simulink model "mission_server_waypoint_qball2"  (Simulink 8.3)
settings: Solver=FixedStepDiscrete  StartTime=0.0  StopTime=inf  FixedStep=0.002  RelTol=1e-3
libraries: quarc_library x6, Orientation_Library x2, simulink x1
settings Model: Creator=CFulford  LastModifiedBy=user  SimulationMode=external  ExtModeTrigDuration=5000
settings SolverCC: PositivePriorityOrder=on
settings OptimizationCC: ExpressionDepthLimit=2147483647  InitFltsAndDblsToZero=on
settings DebuggingCC: FcnCallInpInsideContextMsg=UseLocalSettings
settings SFSimCC: SimParseCustomCode=off
settings RTWCC: SystemTargetFile=quarc_win64.tlc  TemplateMakefile=quarc_default_tmf  Description=QUARC Win64 Target  ProcessScript=quarc_win64_make_rtw_hook
settings STFCustomTargetCC: TargetPreCompLibLocation=C:\PROGRA~3\QUARC\lib\2014a\win64\release  CodeReplacementLibrary=C89/C90 (ANSI)  ConcurrentExecutionCompliant=on  GeneratePreprocessorConditionals=Disable all  CombineOutputUpdateFcns=on  CPPClassGenCompliant=on  GRTInterface=off  SystemTargetFile=quarc_win64.tlc
settings GRTTargetCC: TargetPreCompLibLocation=C:\PROGRA~3\QUARC\lib\2014a\win64\release  CodeReplacementLibrary=C89/C90 (ANSI)  ParMdlRefBuildCompliant=off  CompOptLevelCompliant=off  CombineOutputUpdateFcns=on  MatFileLogging=off  GRTInterface=off  ExtMode=on  ExtModeMexFile=quarc_comm  ExtModeMexArgs='-w -d %d -uri %u','shmem://%m:1?timeout=10'

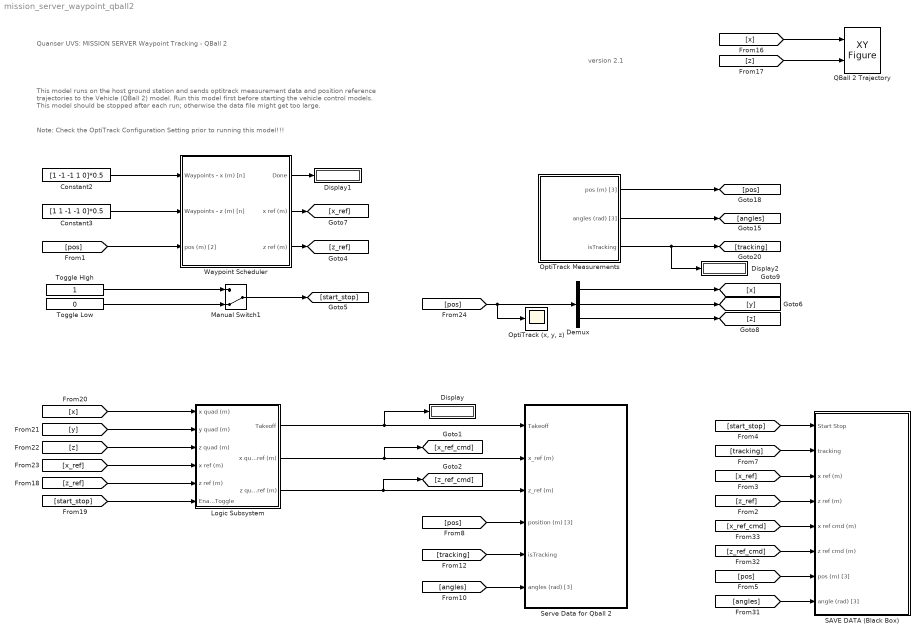
== system mission_server_waypoint_qball2 ==
  note: version 2.1
  note: This model runs on the host ground station and sends
      | optitrack measurement data and position reference trajectories to the Vehicle (QBall 2) model.
      | Run this model first before starting the vehicle control models.
      | This model should be stopped after each run; otherwise the data file might get too large.
  note: Quanser UVS: MISSION SERVER Waypoint Tracking - QBall 2
  note: Note: Check the OptiTrack Configuration Setting prior to running this model!!!
  Constant2 : Constant  Value=[1 -1 -1 1 0]*0.5
  Constant3 : Constant  Value=[1 1 -1 -1 0]*0.5
  Demux : Demux  Outputs=3
  Display : Display
  Display1 : Display
  Display2 : Display
  Logic Subsystem : Subsystem
  Manual Switch1 : ManualSwitch  CurrentSetting=0
  "OptiTrack (x, y, z)" : Scope
      settings: YMin=-0.1  YMax=1.05
  OptiTrack Measurements : Subsystem
  QBall 2 Trajectory : quarc_library/Sinks/Figures/XY Figure  figure_mode=Use figure window  figure_tag=figure1  axes_tag=axes1  minimum_x=-1  maximum_x=1  minimum_y=-1  maximum_y=1  trace_mode=Do not erase old trace  buffer_size=1000  update_rate=100  initial_position="601   63  713  540"  initial_visibility=off  sample_time=-1
  SAVE DATA (Black Box) : Subsystem
  Serve Data for Qball 2 : Subsystem
  Toggle High : Constant
  Toggle Low : Constant  Value=0
  Waypoint Scheduler : Subsystem
  wires:
  [x] -> QBall 2 Trajectory/1
  [z] -> QBall 2 Trajectory/2
  Toggle High/1 -> Manual Switch1/1
  Toggle Low/1 -> Manual Switch1/2
  Manual Switch1/1 -> [start_stop]
  [start_stop] -> Logic Subsystem/6(Enable Toggle)
  [x] -> Logic Subsystem/1(x quad (m))
  [z_ref] -> Logic Subsystem/5(z ref (m))
  [y] -> Logic Subsystem/2(y quad (m))
  [z] -> Logic Subsystem/3(z quad (m))
  [x_ref] -> Logic Subsystem/4(x ref (m))
  Demux/1 -> [x]
  Demux/2 -> [y]
  Demux/3 -> [z]
  OptiTrack Measurements/1(pos (m) [3]) -> [pos]
  OptiTrack Measurements/2(angles (rad) [3]) -> [angles]
  [pos] -> "OptiTrack (x, y, z)"/1, Demux/1
  Logic Subsystem/3(z quad ref (m)) -> [z_ref_cmd], Serve Data for Qball 2/3(z_ref (m))
  Logic Subsystem/1(Takeoff) -> Display/1, Serve Data for Qball 2/1(Takeoff)
  Logic Subsystem/2(x quad ref (m)) -> [x_ref_cmd], Serve Data for Qball 2/2(x_ref (m))
  [tracking] -> Serve Data for Qball 2/5(isTracking)
  [angles] -> Serve Data for Qball 2/6(angles (rad) [3])
  [pos] -> Serve Data for Qball 2/4(position (m) [3])
  OptiTrack Measurements/3(isTracking) -> Display2/1, [tracking]
  Constant3/1 -> Waypoint Scheduler/2(Waypoints - z (m) [n])
  Constant2/1 -> Waypoint Scheduler/1(Waypoints - x (m) [n])
  Waypoint Scheduler/1(Done) -> Display1/1
  Waypoint Scheduler/3(z ref (m)) -> [z_ref]
  Waypoint Scheduler/2(x ref (m)) -> [x_ref]
  [pos] -> Waypoint Scheduler/3(pos (m) [2])
  [z_ref] -> SAVE DATA (Black Box)/4(z ref (m))
  [start_stop] -> SAVE DATA (Black Box)/1(Start Stop)
  [x_ref] -> SAVE DATA (Black Box)/3(x ref (m))
  [pos] -> SAVE DATA (Black Box)/7(pos (m) [3])
  [angles] -> SAVE DATA (Black Box)/8(angle (rad) [3])
  [tracking] -> SAVE DATA (Black Box)/2(tracking)
  [z_ref_cmd] -> SAVE DATA (Black Box)/6(z ref cmd (m))
  [x_ref_cmd] -> SAVE DATA (Black Box)/5(x ref cmd (m))

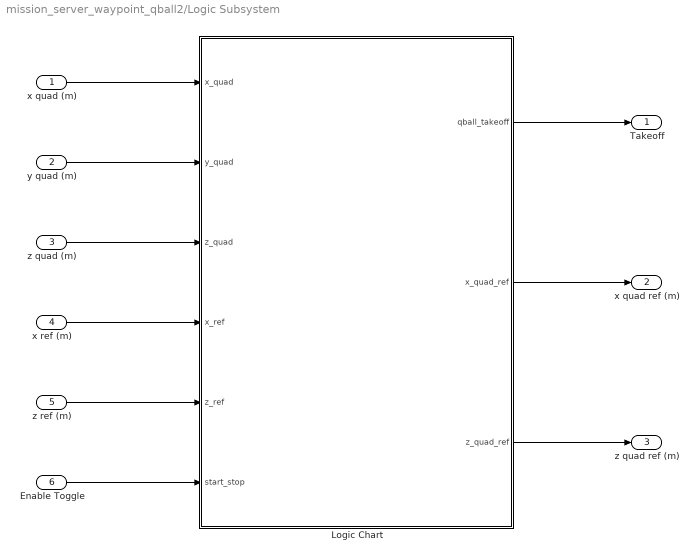
== system mission_server_waypoint_qball2/Logic Subsystem ==
  x quad (m) : Inport
  y quad (m) : Inport  Port=2
  z quad (m) : Inport  Port=3
  x ref (m) : Inport  Port=4
  z ref (m) : Inport  Port=5
  Enable Toggle : Inport  Port=6
  Logic Chart : Stateflow chart  TreatAsAtomicUnit=on
  Takeoff : Outport
  x quad ref (m) : Outport  Port=2
  z quad ref (m) : Outport  Port=3
  wires:
  Logic Chart/2(x_quad_ref) -> x quad ref (m)/1
  Logic Chart/1(qball_takeoff) -> Takeoff/1
  Logic Chart/3(z_quad_ref) -> z quad ref (m)/1
  x quad (m)/1 -> Logic Chart/1(x_quad)
  y quad (m)/1 -> Logic Chart/2(y_quad)
  z quad (m)/1 -> Logic Chart/3(z_quad)
  Enable Toggle/1 -> Logic Chart/6(start_stop)
  x ref (m)/1 -> Logic Chart/4(x_ref)
  z ref (m)/1 -> Logic Chart/5(z_ref)

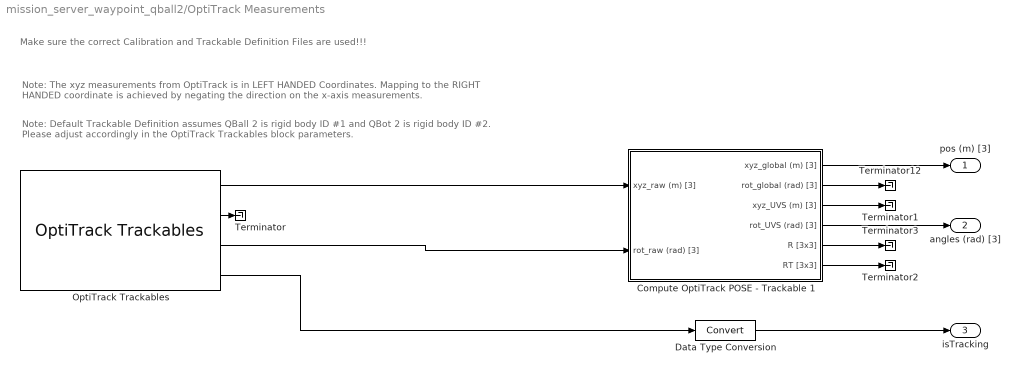
== system mission_server_waypoint_qball2/OptiTrack Measurements ==
  note: Note: The xyz measurements from OptiTrack is in LEFT HANDED Coordinates.
      |
      | Mapping to the RIGHT HANDED coordinate is achieved by negating the direction on the x-axis measurements.
  note: Make sure the correct Calibration and Trackable Definition Files are used!!!
  note: Note: Default Trackable Definition assumes QBall 2 is rigid body ID #1 and QBot 2 is rigid body ID #2.
      | Please adjust accordingly in the OptiTrack Trackables block parameters.
  "Compute OptiTrack POSE - Trackable 1 " : Subsystem
  Data Type Conversion : DataTypeConversion
  OptiTrack Trackables : quarc_library/Devices/Third-Party/NaturalPoint/OptiTrack/OptiTrack Trackables  calibration_file=C:\Users\user\Desktop\final\Calibration Very High Quality Exceptional (MeanErr 0.001 mm) 2017-05-16 6.48pm.cal  rigid_body_file=C:\Users\user\Desktop\final\RigidBodies 2017-05-26 7.29pm.tra  rigid_body_ids=[1]  sample_time=qc_get_step_size
  Terminator{,1..3,12} (5 alike) : Terminator
  pos (m) [3] : Outport
  angles (rad) [3] : Outport  Port=2
  isTracking : Outport  Port=3
  wires:
  OptiTrack Trackables/4 -> Data Type Conversion/1
  OptiTrack Trackables/2 -> Terminator/1
  "Compute OptiTrack POSE - Trackable 1 "/1(xyz_global (m) [3]) -> pos (m) [3]/1
  "Compute OptiTrack POSE - Trackable 1 "/4(rot_UVS (rad) [3]) -> angles (rad) [3]/1
  "Compute OptiTrack POSE - Trackable 1 "/3(xyz_UVS (m) [3]) -> Terminator1/1
  "Compute OptiTrack POSE - Trackable 1 "/2(rot_global (rad) [3]) -> Terminator12/1
  "Compute OptiTrack POSE - Trackable 1 "/5(R [3x3]) -> Terminator3/1
  "Compute OptiTrack POSE - Trackable 1 "/6(RT [3x3]) -> Terminator2/1
  OptiTrack Trackables/1 -> "Compute OptiTrack POSE - Trackable 1 "/1(xyz_raw (m) [3])
  OptiTrack Trackables/3 -> "Compute OptiTrack POSE - Trackable 1 "/2(rot_raw (rad) [3])
  Data Type Conversion/1 -> isTracking/1

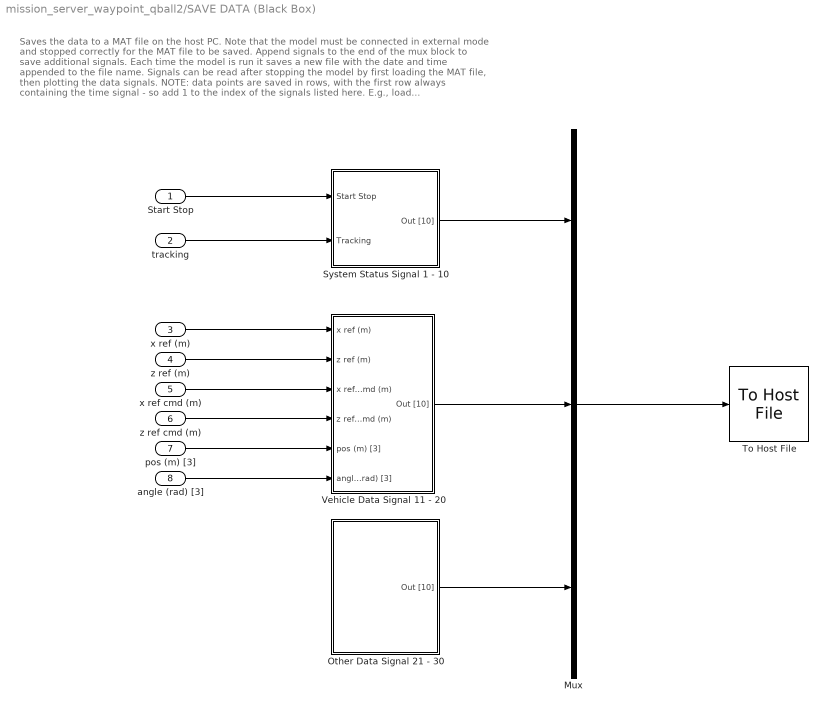
== system mission_server_waypoint_qball2/SAVE DATA (Black Box) ==
  note: Saves the data to a MAT file on the host PC. Note that the model must be connected
      | in external mode and stopped correctly for the MAT file to be saved.
      | Append signals to the end of the mux block to save additional signals.
      | Each time the model is run it saves a new file with the date and time appended
      | to the file name.
      |
      | Signals can be read after stopping the model by first loading the MAT file, then plotting
      | the data signals. NOTE: data points are saved in rows, with the first row always containing
      | the time signal - so add 1 to the index of the signals listed here. E.g.,
      |
      | load mission_data.mat
      | t = mission_data(1,:);
      | roll = mission_data(22,:);
      | plot(t, roll);
  Start Stop : Inport
  tracking : Inport  Port=2
  x ref (m) : Inport  Port=3
  z ref (m) : Inport  Port=4
  x ref cmd (m) : Inport  Port=5
  z ref cmd (m) : Inport  Port=6
  pos (m) [3] : Inport  Port=7
  angle (rad) [3] : Inport  Port=8
  Mux : Mux  Inputs=3
  Other Data Signal 21 - 30 : Subsystem
  System Status Signal 1 - 10 : Subsystem
  To Host File : quarc_library/Sinks/To Host/To Host File  file_name=mission_data_%{date}_%{time}.mat  variable_name=mission_data  decimation=1  sample_time=-1  file_format=MAT-file v.4  options=No header or footer  append=off  final_file_name=mission_data_26-May-2017_19-37-20.mat
  Vehicle Data Signal 11 - 20 : Subsystem
  wires:
  Start Stop/1 -> System Status Signal 1 - 10/1(Start Stop)
  tracking/1 -> System Status Signal 1 - 10/2(Tracking)
  z ref (m)/1 -> Vehicle Data Signal 11 - 20/2(z ref (m))
  x ref (m)/1 -> Vehicle Data Signal 11 - 20/1(x ref (m))
  pos (m) [3]/1 -> Vehicle Data Signal 11 - 20/5(pos (m) [3])
  angle (rad) [3]/1 -> Vehicle Data Signal 11 - 20/6(angle (rad) [3])
  System Status Signal 1 - 10/1(Out [10]) -> Mux/1
  Vehicle Data Signal 11 - 20/1(Out [10]) -> Mux/2
  Other Data Signal 21 - 30/1(Out [10]) -> Mux/3
  Mux/1 -> To Host File/1
  z ref cmd (m)/1 -> Vehicle Data Signal 11 - 20/4(z ref cmd (m))
  x ref cmd (m)/1 -> Vehicle Data Signal 11 - 20/3(x ref cmd (m))

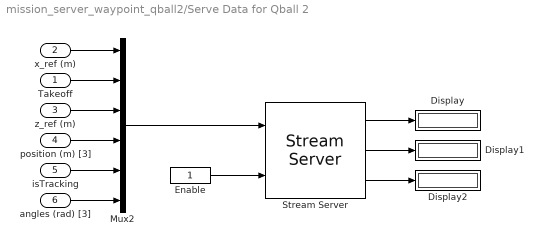
== system mission_server_waypoint_qball2/Serve Data for Qball 2 ==
  Takeoff : Inport
  x_ref (m) : Inport  Port=2
  z_ref (m) : Inport  Port=3
  position (m) [3] : Inport  Port=4
  isTracking : Inport  Port=5
  angles (rad) [3] : Inport  Port=6
  Display : Display
      settings: Decimation=100
  Display1 : Display
      settings: Decimation=100
  Display2 : Display
      settings: Decimation=100
  Enable : Constant
  Mux2 : Mux  Inputs=[1 1 1 3 1 3]
  Stream Server : quarc_library/Communications/Basic/Stream Server  uri_source=Specify via dialog (do not evaluate)  uri=tcpip://localhost:18006  apply_uri_to_all_configs=on  send_buffer_size=1460  receive_buffer_size=1460  byte_order=little endian (Intel - LSB first)  optimization=Minimum latency  implementation=Use non-blocking I/O  send_options=Send most recent data  receive_options=Do not receive data  send_fifo_size=1000  receive_fifo_size=1000  send_priority=0  receive_priority=0  default_value=[0]  send_dimensions=off  receive_dimensions=off  max_dimensions=-1  sample_time=qc_get_step_size  active=off  data_type=Inherited via back propagation  type_expr=BusObject
      settings: AttributesFormatString="\"tcpip://localhost:18006\""
  wires:
  Enable/1 -> Stream Server/2
  Stream Server/1 -> Display/1
  Stream Server/2 -> Display1/1
  Stream Server/3 -> Display2/1
  z_ref (m)/1 -> Mux2/3
  position (m) [3]/1 -> Mux2/4
  Takeoff/1 -> Mux2/2
  isTracking/1 -> Mux2/5
  x_ref (m)/1 -> Mux2/1
  angles (rad) [3]/1 -> Mux2/6
  Mux2/1 -> Stream Server/1

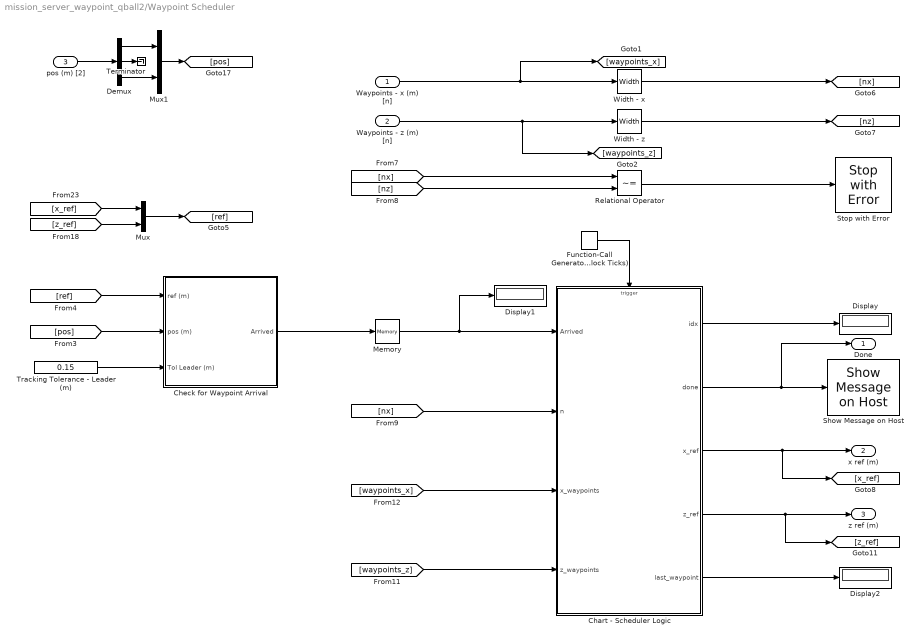
== system mission_server_waypoint_qball2/Waypoint Scheduler ==
  Waypoints - x (m) [n] : Inport
  Waypoints - z (m) [n] : Inport  Port=2
  pos (m) [2] : Inport  Port=3
  Chart - Scheduler Logic : Stateflow chart  TreatAsAtomicUnit=on
  Check for Waypoint Arrival : Subsystem
  Demux : Demux  Outputs=3
  Display : Display
      settings: Decimation=100
  Display1 : Display
      settings: Decimation=100
  Display2 : Display
      settings: Decimation=100
  Function-Call Generator (Clock Ticks) : simulink/Ports & Subsystems/Function-Call Generator  sample_time=qc_get_step_size  numberOfIterations=1
  Memory : Memory
  Mux : Mux  Inputs=2
  Mux1 : Mux  Inputs=2
  Relational Operator : RelationalOperator  Operator=~=  OutDataTypeStr=boolean
  Show Message on Host : quarc_library/Sinks/Error Handling/Show Message on Host  message_type=Fixed error message  message_icon=Information  message=Vehicles at final waypoint. Please land QBall and then stop all models.
      settings: AttributesFormatString="\"%<message>\""
  Stop with Error : quarc_library/Sinks/Error Handling/Stop with Error  message_type=Fixed error message  message=Error: Number of x and z waypoints not equal!
      settings: AttributesFormatString="\"%<message>\""
  Terminator : Terminator
  Tracking Tolerance - Leader (m) : Constant  Value=0.15
  Width - x : Width
  Width - z : Width
  Done : Outport
  x ref (m) : Outport  Port=2
  z ref (m) : Outport  Port=3
  wires:
  Waypoints - x (m) [n]/1 -> Width - x/1, [waypoints_x]
  Waypoints - z (m) [n]/1 -> Width - z/1, [waypoints_z]
  [x_ref] -> Mux/1
  [z_ref] -> Mux/2
  Mux/1 -> [ref]
  Width - x/1 -> [nx]
  Width - z/1 -> [nz]
  [nx] -> Relational Operator/1
  [nz] -> Relational Operator/2
  Relational Operator/1 -> Stop with Error/1
  Chart - Scheduler Logic/3(x_ref) -> [x_ref], x ref (m)/1
  Chart - Scheduler Logic/4(z_ref) -> [z_ref], z ref (m)/1
  Chart - Scheduler Logic/2(done) -> Done/1, Show Message on Host/1
  Chart - Scheduler Logic/1(idx) -> Display/1
  Function-Call Generator (Clock Ticks)/1 -> Chart - Scheduler Logic/Trigger
  [nx] -> Chart - Scheduler Logic/2(n)
  [waypoints_x] -> Chart - Scheduler Logic/3(x_waypoints)
  [waypoints_z] -> Chart - Scheduler Logic/4(z_waypoints)
  [ref] -> Check for Waypoint Arrival/1(ref (m))
  [pos] -> Check for Waypoint Arrival/2(pos (m))
  Check for Waypoint Arrival/1(Arrived) -> Memory/1
  Memory/1 -> Display1/1, Chart - Scheduler Logic/1(Arrived)
  pos (m) [2]/1 -> Demux/1
  Demux/1 -> Mux1/1
  Demux/3 -> Mux1/2
  Mux1/1 -> [pos]
  Demux/2 -> Terminator/1
  Tracking Tolerance - Leader (m)/1 -> Check for Waypoint Arrival/3(Tol Leader (m))
  Chart - Scheduler Logic/5(last_waypoint) -> Display2/1

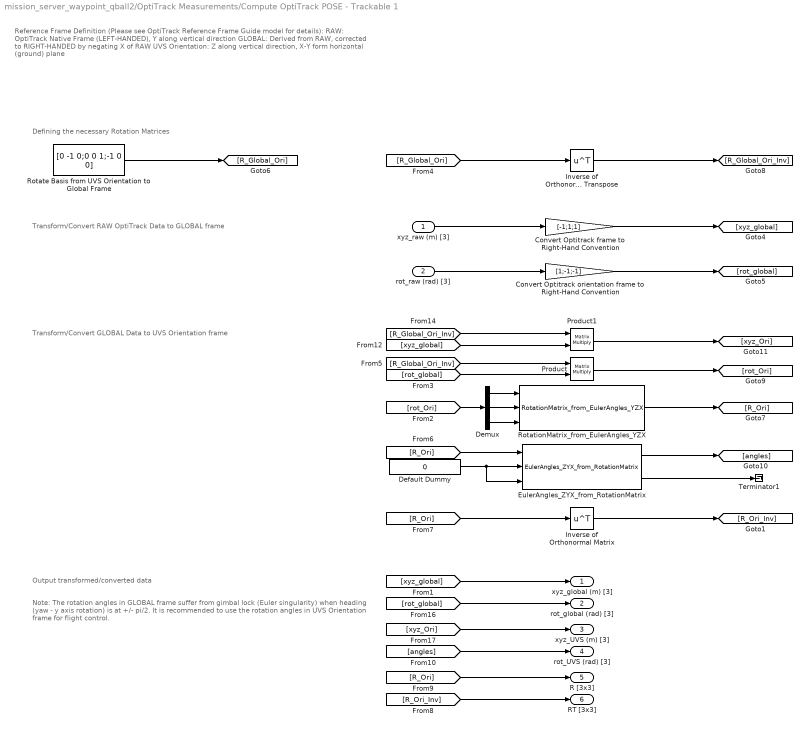
== system mission_server_waypoint_qball2/OptiTrack Measurements/Compute OptiTrack POSE - Trackable 1  ==
  note: Transform/Convert RAW OptiTrack Data to GLOBAL frame
  note: Defining the necessary Rotation Matrices
  note: Reference Frame Definition (Please see OptiTrack Reference Frame Guide model for details):
      |
      | RAW: OptiTrack Native Frame (LEFT-HANDED), Y along vertical direction
      | GLOBAL: Derived from RAW, corrected to RIGHT-HANDED by negating X of RAW
      | UVS Orientation: Z along vertical direction, X-Y form horizontal (ground) plane
  note: Transform/Convert GLOBAL Data to UVS Orientation frame
  note: Output transformed/converted data
  note: Note: The rotation angles in GLOBAL frame suffer from gimbal lock (Euler singularity)
      | when heading (yaw - y axis rotation) is at +/- pi/2.
      | It is recommended to use the rotation angles in UVS Orientation frame for flight control.
  xyz_raw (m) [3] : Inport
  rot_raw (rad) [3] : Inport  Port=2
  Convert Optitrack frame to Right-Hand Convention : Gain  Gain=[-1;1;1]
  Convert Optitrack orientation frame to Right-Hand Convention : Gain  Gain=[1;-1;-1]
  Default Dummy : Constant  Value=0
  Demux : Demux  Outputs=3
  EulerAngles_ZYX_from_RotationMatrix : Orientation_Library/EulerAngles_ZYX_from_RotationMatrix
  Inverse of Orthonormal Matrix : Math  Operator=transpose  SaturateOnIntegerOverflow=on
  Inverse of Orthonormal Matrix is its Transpose : Math  Operator=transpose  SaturateOnIntegerOverflow=on
  Product : Product  Multiplication=Matrix(*)
  Product1 : Product  Multiplication=Matrix(*)
  Rotate Basis from UVS Orientation to Global Frame : Constant  Value=[0 -1 0;0 0 1;-1 0 0]
  RotationMatrix_from_EulerAngles_YZX : Orientation_Library/RotationMatrix_from_EulerAngles_YZX
  Terminator1 : Terminator
  xyz_global (m) [3] : Outport
  rot_global (rad) [3] : Outport  Port=2
  xyz_UVS (m) [3] : Outport  Port=3
  rot_UVS (rad) [3] : Outport  Port=4
  R [3x3] : Outport  Port=5
  RT [3x3] : Outport  Port=6
  wires:
  Rotate Basis from UVS Orientation to Global Frame/1 -> [R_Global_Ori]
  [R_Global_Ori] -> Inverse of Orthonormal Matrix is its Transpose/1
  Inverse of Orthonormal Matrix is its Transpose/1 -> [R_Global_Ori_Inv]
  Convert Optitrack orientation frame to Right-Hand Convention/1 -> [rot_global]
  xyz_raw (m) [3]/1 -> Convert Optitrack frame to Right-Hand Convention/1
  Convert Optitrack frame to Right-Hand Convention/1 -> [xyz_global]
  rot_raw (rad) [3]/1 -> Convert Optitrack orientation frame to Right-Hand Convention/1
  [R_Global_Ori_Inv] -> Product1/1
  [xyz_global] -> Product1/2
  Product1/1 -> [xyz_Ori]
  [R_Global_Ori_Inv] -> Product/1
  Product/1 -> [rot_Ori]
  [rot_global] -> Product/2
  [rot_Ori] -> Demux/1
  Demux/1 -> RotationMatrix_from_EulerAngles_YZX/1
  Demux/2 -> RotationMatrix_from_EulerAngles_YZX/2
  RotationMatrix_from_EulerAngles_YZX/1 -> [R_Ori]
  Demux/3 -> RotationMatrix_from_EulerAngles_YZX/3
  [R_Ori] -> EulerAngles_ZYX_from_RotationMatrix/1
  Default Dummy/1 -> EulerAngles_ZYX_from_RotationMatrix/3, EulerAngles_ZYX_from_RotationMatrix/2
  EulerAngles_ZYX_from_RotationMatrix/2 -> Terminator1/1
  EulerAngles_ZYX_from_RotationMatrix/1 -> [angles]
  [xyz_global] -> xyz_global (m) [3]/1
  [rot_global] -> rot_global (rad) [3]/1
  [xyz_Ori] -> xyz_UVS (m) [3]/1
  [angles] -> rot_UVS (rad) [3]/1
  [R_Ori] -> Inverse of Orthonormal Matrix/1
  Inverse of Orthonormal Matrix/1 -> [R_Ori_Inv]
  [R_Ori] -> R [3x3]/1
  [R_Ori_Inv] -> RT [3x3]/1

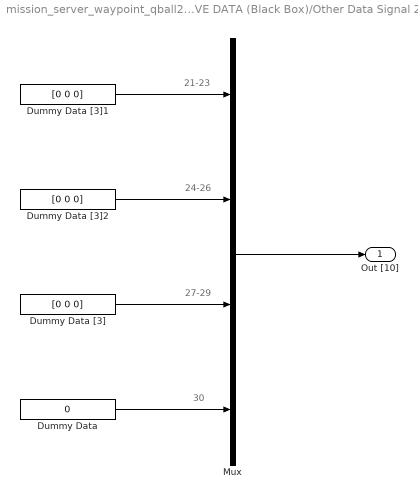
== system mission_server_waypoint_qball2/SAVE DATA (Black Box)/Other Data Signal 21 - 30 ==
  note: 30
  note: 27-29
  note: 24-26
  note: 21-23
  Dummy Data : Constant  Value=0
  Dummy Data [3] : Constant  Value=[0 0 0]
  Dummy Data [3]1 : Constant  Value=[0 0 0]
  Dummy Data [3]2 : Constant  Value=[0 0 0]
  Mux : Mux  Inputs=[3 3 3 1]
  Out [10] : Outport
  wires:
  Mux/1 -> Out [10]/1
  Dummy Data [3]/1 -> Mux/3
  Dummy Data/1 -> Mux/4
  Dummy Data [3]1/1 -> Mux/1
  Dummy Data [3]2/1 -> Mux/2

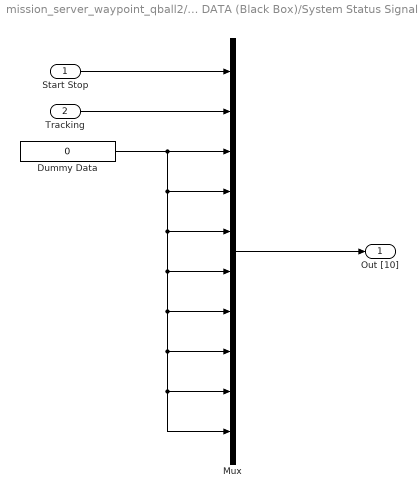
== system mission_server_waypoint_qball2/SAVE DATA (Black Box)/System Status Signal 1 - 10 ==
  Start Stop : Inport
  Tracking : Inport  Port=2
  Dummy Data : Constant  Value=0
  Mux : Mux  Inputs=10
  Out [10] : Outport
  wires:
  Tracking/1 -> Mux/2
  Start Stop/1 -> Mux/1
  Dummy Data/1 -> Mux/3, Mux/7, Mux/8, Mux/9, Mux/10, Mux/6, Mux/5, Mux/4
  Mux/1 -> Out [10]/1

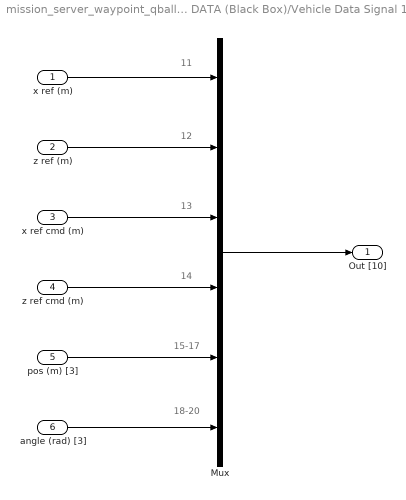
== system mission_server_waypoint_qball2/SAVE DATA (Black Box)/Vehicle Data Signal 11 - 20 ==
  note: 11
  note: 12
  note: 13
  note: 15-17
  note: 14
  note: 18-20
  x ref (m) : Inport
  z ref (m) : Inport  Port=2
  x ref cmd (m) : Inport  Port=3
  z ref cmd (m) : Inport  Port=4
  pos (m) [3] : Inport  Port=5
  angle (rad) [3] : Inport  Port=6
  Mux : Mux  Inputs=[1 1 1 1 3 3]
  Out [10] : Outport
  wires:
  Mux/1 -> Out [10]/1
  x ref (m)/1 -> Mux/1
  z ref (m)/1 -> Mux/2
  x ref cmd (m)/1 -> Mux/3
  z ref cmd (m)/1 -> Mux/4
  pos (m) [3]/1 -> Mux/5
  angle (rad) [3]/1 -> Mux/6

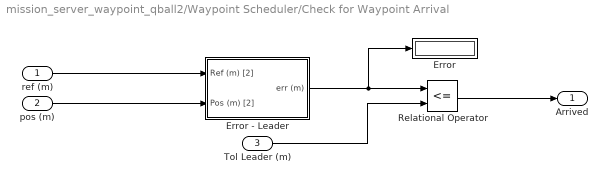
== system mission_server_waypoint_qball2/Waypoint Scheduler/Check for Waypoint Arrival ==
  ref (m) : Inport
  pos (m) : Inport  Port=2
  Tol Leader (m) : Inport  Port=3
  Error : Display
  Error - Leader : Subsystem
  Relational Operator : RelationalOperator  Operator=<=  OutDataTypeStr=boolean
  Arrived : Outport
  wires:
  pos (m)/1 -> Error - Leader/2(Pos (m) [2])
  ref (m)/1 -> Error - Leader/1(Ref (m) [2])
  Error - Leader/1(err (m)) -> Error/1, Relational Operator/1
  Tol Leader (m)/1 -> Relational Operator/2
  Relational Operator/1 -> Arrived/1

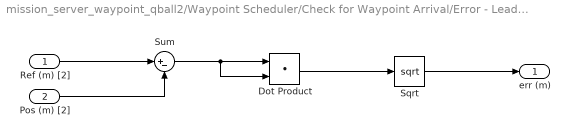
== system mission_server_waypoint_qball2/Waypoint Scheduler/Check for Waypoint Arrival/Error - Leader ==
  Ref (m) [2] : Inport
  Pos (m) [2] : Inport  Port=2
  Dot Product : DotProduct  InputSameDT=on  OutDataTypeStr=Inherit: Inherit via internal rule
  Sqrt : Sqrt  SaturateOnIntegerOverflow=on
  Sum : Sum  Inputs=|+-
  err (m) : Outport
  wires:
  Ref (m) [2]/1 -> Sum/1
  Pos (m) [2]/1 -> Sum/2
  Sum/1 -> Dot Product/2, Dot Product/1
  Dot Product/1 -> Sqrt/1
  Sqrt/1 -> err (m)/1

== stateflow chart Logic Subsystem/Logic Chart ==
  state WaitForStartCommand
    du:
    qball_takeoff = 0
    x_quad_ref = x_quad
    z_quad_ref = z_quad
  state Takeoff
    entry:
    qball_takeoff = 1
  state QballGetsWaypoints
    du:
    x_quad_ref = x_ref
    z_quad_ref = z_ref
  state Landing
    entry:
    qball_takeoff=0;
    x_quad_ref=x_quad;
    z_quad_ref=z_quad;
  (default) -> WaitForStartCommand
  WaitForStartCommand -> Takeoff : [hasChanged(start_stop)]
  Takeoff -> QballGetsWaypoints [order 1] : [y_quad >= MIN_QUAD_HEIGHT]
  Takeoff -> Landing [order 2] : [hasChanged(start_stop)]
  QballGetsWaypoints -> Landing : [hasChanged(start_stop)]
  data: qball_takeoff output double =0; x_quad input double; y_quad input double; z_quad input double; x_ref input double; z_ref input double; x_quad_ref output double; z_quad_ref output double; start_stop input double; MIN_QUAD_HEIGHT constant double =0.5

== stateflow chart Waypoint Scheduler/Chart - Scheduler Logic ==
  state Increment_Index
    entry:
    if(idx==n)
    done=1;
    else
    idx = idx+1;
    end;
  state Issue_CMD
    entry:
    if(idx==n)
    last_waypoint = 1;
    end;
    during:
    x_ref = x_waypoints(idx);
    z_ref = z_waypoints(idx);
  state Init
    entry:
    done = 0;
    idx = 1;
    last_waypoint=0;
    x_ref = x_waypoints(idx);
    z_ref = z_waypoints(idx);
  Issue_CMD -> Increment_Index : after(1, sec)[Arrived==1]
  Init -> Issue_CMD
  (default) -> Init
  Increment_Index -> Issue_CMD
  data: idx output double [0..]; done output double [0..1]; x_ref output double; z_ref output double; Arrived input double [0..1]; n input double; x_waypoints input double; z_waypoints input double; last_waypoint output double [0..1]
  events: tick input FUNCTION_CALL_EVENT
